simulink library "actuator_S2_lib"  (Simulink 6.6)
libraries: aeroutilslib x8, simulink x1
settings Model: Creator=amurch  LastModifiedBy=amurch

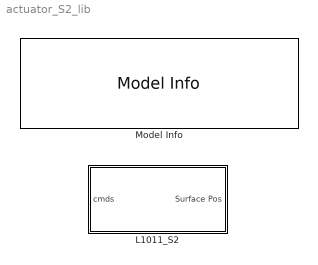
== system actuator_S2_lib ==
  L1011_S2 : Subsystem
  Model Info : simulink/Model-Wide Utilities/Model Info  SystemSampleTime=-1  InitialBlockCM=None  BlockCM=None  Frame=on  DisplayStringWithTags=|  HorizontalTextAlignment=Center  LeftAlignmentValue=0.5  SourceBlockDiagram=actuator_S2_lib  TagMaxNumber=20
      | Actuator Library
      | %<ModelVersion>
      | Las modified by %<LastModifiedBy> on %<LastModificationDate>

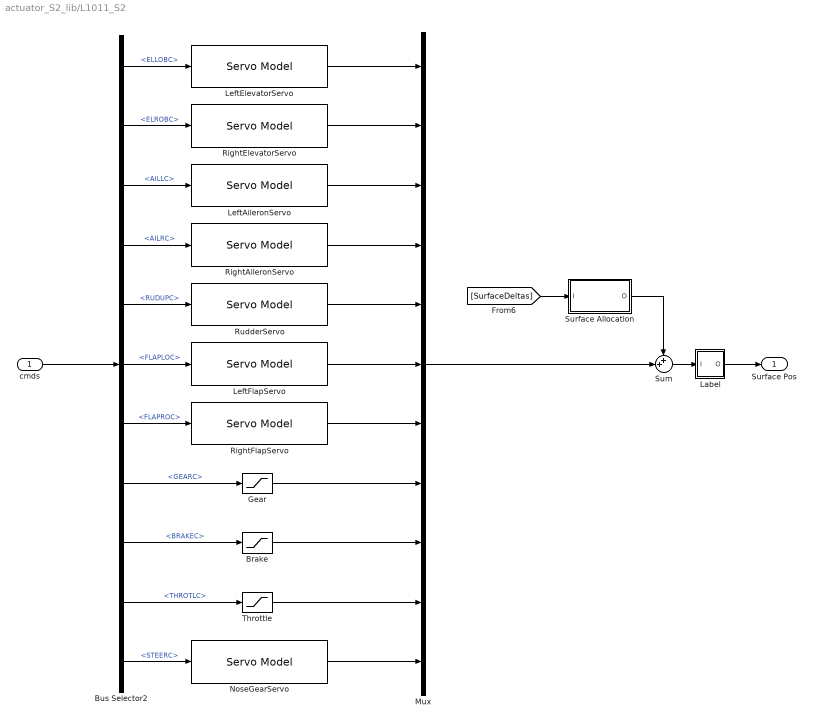
== system actuator_S2_lib/L1011_S2 ==
  cmds : Inport
  Brake : Saturate  UpperLimit=1.0  LowerLimit=0.0
  Bus Selector2 : BusSelector  OutputSignals=ELLOBC,ELROBC,AILLC,AILRC,RUDUPC,FLAPLOC,FLAPROC,GEARC,BRAKEC,THROTLC,STEERC
  Gear : Saturate  UpperLimit=1.0  LowerLimit=0.0
  Label : Subsystem
  LeftAileronServo : aeroutilslib/Servo Model  SystemSampleTime=-1  freq=10  RL=300  POS_hi=20  POS_lo=-20
  LeftElevatorServo : aeroutilslib/Servo Model  SystemSampleTime=-1  freq=10  RL=300  POS_hi=20  POS_lo=-30
  LeftFlapServo : aeroutilslib/Servo Model  SystemSampleTime=-1  freq=10  RL=300  POS_hi=45  POS_lo=0
  Mux : Mux  Inputs=11
  NoseGearServo : aeroutilslib/Servo Model  SystemSampleTime=-1  freq=10  RL=300  POS_hi=30  POS_lo=-30
  RightAileronServo : aeroutilslib/Servo Model  SystemSampleTime=-1  freq=10  RL=300  POS_hi=20  POS_lo=-20
  RightElevatorServo : aeroutilslib/Servo Model  SystemSampleTime=-1  freq=10  RL=300  POS_hi=20  POS_lo=-30
  RightFlapServo : aeroutilslib/Servo Model  SystemSampleTime=-1  freq=10  RL=300  POS_hi=45  POS_lo=0
  RudderServo : aeroutilslib/Servo Model  SystemSampleTime=-1  freq=8.4  RL=300  POS_hi=30  POS_lo=-30.0
  Sum : Sum  Inputs=++|
  Surface Allocation : Subsystem
  Throttle : Saturate  UpperLimit=100  LowerLimit=0.0
  Surface Pos : Outport
  wires:
  Surface Allocation/1(O) -> Sum/1
  cmds/1 -> Bus Selector2/1
  [SurfaceDeltas] -> Surface Allocation/1(I)
  Label/1(O) -> Surface Pos/1
  Sum/1 -> Label/1(I)
  Mux/1 -> Sum/2
  LeftElevatorServo/1 -> Mux/1
  RightElevatorServo/1 -> Mux/2
  LeftAileronServo/1 -> Mux/3
  RightAileronServo/1 -> Mux/4
  RudderServo/1 -> Mux/5
  LeftFlapServo/1 -> Mux/6
  RightFlapServo/1 -> Mux/7
  Gear/1 -> Mux/8
  Brake/1 -> Mux/9
  Throttle/1 -> Mux/10
  Bus Selector2/1 -> LeftElevatorServo/1  "<ELLOBC>"
  Bus Selector2/2 -> RightElevatorServo/1  "<ELROBC>"
  Bus Selector2/3 -> LeftAileronServo/1  "<AILLC>"
  Bus Selector2/4 -> RightAileronServo/1  "<AILRC>"
  Bus Selector2/5 -> RudderServo/1  "<RUDUPC>"
  Bus Selector2/6 -> LeftFlapServo/1  "<FLAPLOC>"
  Bus Selector2/7 -> RightFlapServo/1  "<FLAPROC>"
  Bus Selector2/8 -> Gear/1  "<GEARC>"
  Bus Selector2/9 -> Brake/1  "<BRAKEC>"
  Bus Selector2/10 -> Throttle/1  "<THROTLC>"
  Bus Selector2/11 -> NoseGearServo/1  "<STEERC>"
  NoseGearServo/1 -> Mux/11

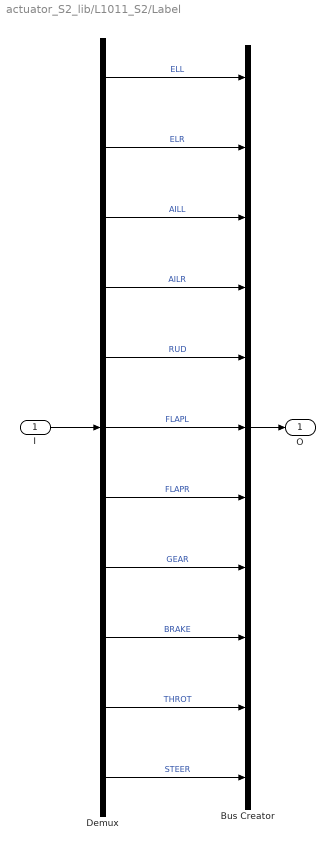
== system actuator_S2_lib/L1011_S2/Label ==
  I : Inport
  Bus Creator : BusCreator  Inputs=11
  Demux : Demux  Outputs=11
  O : Outport
  wires:
  Demux/1 -> Bus Creator/1  "ELL"
  Demux/4 -> Bus Creator/4  "AILR"
  Demux/3 -> Bus Creator/3  "AILL"
  Demux/2 -> Bus Creator/2  "ELR"
  Bus Creator/1 -> O/1
  I/1 -> Demux/1
  Demux/5 -> Bus Creator/5  "RUD"
  Demux/6 -> Bus Creator/6  "FLAPL"
  Demux/7 -> Bus Creator/7  "FLAPR"
  Demux/8 -> Bus Creator/8  "GEAR"
  Demux/9 -> Bus Creator/9  "BRAKE"
  Demux/10 -> Bus Creator/10  "THROT"
  Demux/11 -> Bus Creator/11  "STEER"

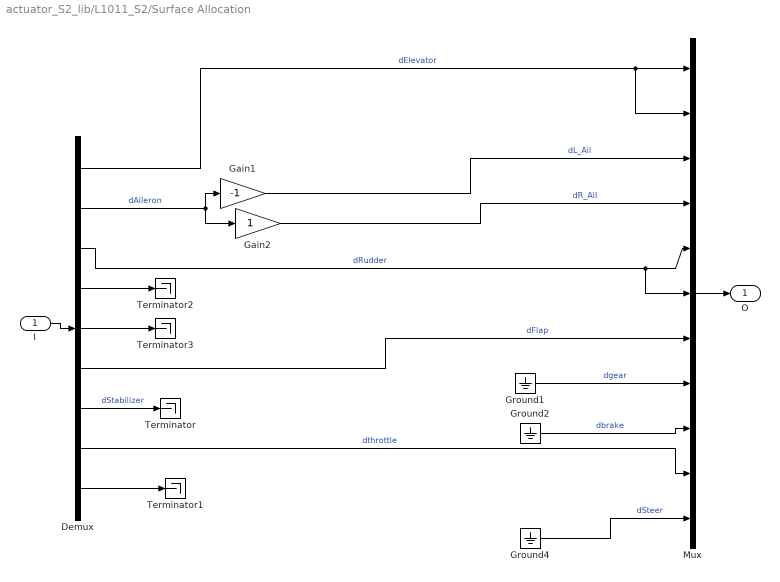
== system actuator_S2_lib/L1011_S2/Surface Allocation ==
  I : Inport
  Demux : Demux  Outputs=9
  Gain1 : Gain  Gain=-1
  Gain2 : Gain
  Ground1 : Ground
  Ground2 : Ground
  Ground4 : Ground
  Mux : Mux  Inputs=11
  Terminator{,1..3} (4 alike) : Terminator
  O : Outport
  wires:
  Mux/1 -> O/1
  Demux/2 -> Gain2/1, Gain1/1  "dAileron"
  I/1 -> Demux/1
  Ground1/1 -> Mux/8  "dgear"
  Ground2/1 -> Mux/9  "dbrake"
  Demux/8 -> Mux/10  "dthrottle"
  Gain1/1 -> Mux/3  "dL_Ail"
  Gain2/1 -> Mux/4  "dR_Ail"
  Demux/3 -> Mux/5, Mux/6  "dRudder"
  Demux/6 -> Mux/7  "dFlap"
  Demux/7 -> Terminator/1  "dStabilizer"
  Demux/1 -> Mux/1, Mux/2  "dElevator"
  Ground4/1 -> Mux/11  "dSteer"
  Demux/4 -> Terminator2/1
  Demux/5 -> Terminator3/1
  Demux/9 -> Terminator1/1
